simulink model "button_test"  (R2013b)
settings: Solver=FixedStepDiscrete  StartTime=0.0  StopTime=200  RelTol=1e-3
undefined symbols (not defined in the file): Green, led0
libraries: embdlinuxlib x2
settings Model: SimulationMode=external  ExtModeTrigDuration=100  Creator=mouyang  LastModifiedBy=mouyang
settings OptimizationCC: OptimizeModelRefInitCode=on  LifeSpan=Inf
settings DebuggingCC: SolverPrmCheckMsg=none
settings HardwareCC: ProdLargestAtomicInteger=Long  ProdLargestAtomicFloat=Double  ProdEndianess=LittleEndian  ProdHWDeviceType=ARM Compatible->ARM Cortex
settings RTWCC: SystemTargetFile=realtime.tlc  GenerateMakefile=off  TemplateMakefile=realtime.tmf  Description=Run on Target Hardware  RTWVerbose=off  ProcessScript=realtime_make_rtw_hook
settings STFCustomTargetCC: TargetLibSuffix=.a  GenerateSampleERTMain=on  ERTCustomFileBanners=on  SupportNonInlinedSFcns=off  SupportVariableSizeSignals=on  MATLABClassNameForMDSCustomization=Simulink.SoftwareTarget.ERTCustomization  GRTInterface=off  SystemTargetFile=realtime.tlc
settings ERTTargetCC: CodeReplacementLibrary=ANSI_C  GenerateSampleERTMain=on  ParMdlRefBuildCompliant=off  CompOptLevelCompliant=off  ConcurrentExecutionCompliant=off  CombineOutputUpdateFcns=off  ERTFirstTimeCompliant=off  SupportContinuousTime=on  SupportVariableSizeSignals=on  ModelStepFunctionPrototypeControlCompliant=off  CPPClassGenCompliant=off  ExtModeMexArgs='192.168.200.24' 0 17725  InlinedParameterPlacement=NonHierarchical  ERTSrcFileBannerTemplate=realtime_code_template.cgt  ERTHdrFileBannerTemplate=realtime_code_template.cgt  ERTDataSrcFileTemplate=realtime_code_template.cgt  ERTDataHdrFileTemplate=realtime_code_template.cgt  ERTCustomFileTemplate=realtime_file_process.tlc

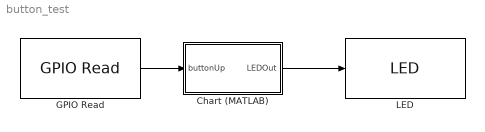
== system button_test ==
  Chart (MATLAB) : Stateflow chart  TreatAsAtomicUnit=on
  GPIO Read : embdlinuxlib/GPIO Read  board=Model B Rev2  gpio=4  internalResistor=Off  sampleTime=0.1  direction=Input  blockPlatform=Raspberry Pi
  LED : embdlinuxlib/LED  board=Model B Rev1  led=led0 (Green)  blockPlatform=Raspberry Pi
  wires:
  GPIO Read/1 -> Chart (MATLAB)/1(buttonUp)
  Chart (MATLAB)/1(LEDOut) -> LED/1

== stateflow chart button_test/Chart (MATLAB) ==
  state init_wait
  state On_state
    en:LEDOut=true;
  state Off_state
    en:LEDOut=false;
  (default) -> init_wait
  init_wait -> On_state : [isequal(buttonUp,false)]
  Off_state -> On_state : [isequal(buttonUp,false)]
  On_state -> Off_state : [isequal(buttonUp,false)]
  data: buttonUp input; LEDOut output boolean
